simulink model "secondpart"  (R2022a)
settings: Solver=FixedStepAuto  StartTime=0.0  StopTime=5  FixedStep=0.2  RelTol=1e-3
settings Model: Creator=P1oruN7  LastModifiedBy=P1oruN7

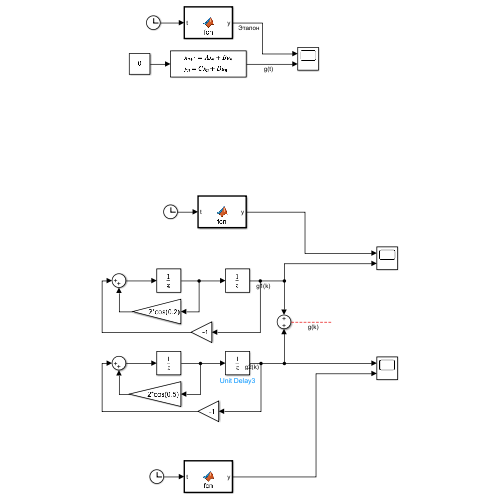
[thumbnail: Simulink's stored preview of the top-level diagram]
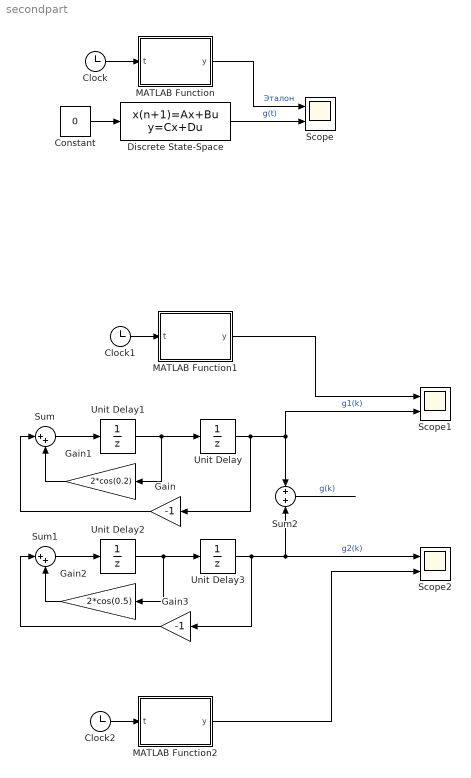
== system secondpart ==
  Clock : Clock
  Clock1 : Clock
  Clock2 : Clock
  Constant : Constant  Value=0
  Discrete State-Space : DiscreteStateSpace  A=[0 1 0 0; -1 2*cos(0.2) 0 0; 0 0 0 1; 0 0 -1 2*cos(0.5)]  B=[1; 1; 1; 1]  C=[1 0 1 0]  D=0  InitialCondition=[0; 8*sin(0.2); 1.5; 1.5*cos(0.5)]  SampleTime=0.2
  Gain : Gain  Gain=-1
  Gain1 : Gain  Gain=2*cos(0.2)
  Gain2 : Gain  Gain=2*cos(0.5)
  Gain3 : Gain  Gain=-1
  MATLAB Function : MATLAB Function  TreatAsAtomicUnit=on
  MATLAB Function1 : MATLAB Function  TreatAsAtomicUnit=on
  MATLAB Function2 : MATLAB Function  TreatAsAtomicUnit=on
  Scope : Scope  NumInputPorts=2
  Scope1 : Scope  NumInputPorts=2
  Scope2 : Scope  NumInputPorts=2
  Sum : Sum  Inputs=|++
  Sum1 : Sum  Inputs=|++
  Sum2 : Sum
  Unit Delay : UnitDelay  SampleTime=-1  HasFrameUpgradeWarning=on
  Unit Delay1 : UnitDelay  InitialCondition=8*sin(0.2)  SampleTime=-1  HasFrameUpgradeWarning=on
  Unit Delay2 : UnitDelay  InitialCondition=1.5*cos(0.5)  SampleTime=-1  HasFrameUpgradeWarning=on
  Unit Delay3 : UnitDelay  SampleTime=-1  HasFrameUpgradeWarning=on
  wires:
  Clock/1 -> MATLAB Function/1(t)
  Constant/1 -> Discrete State-Space/1
  Discrete State-Space/1 -> Scope/2  "g(t)"
  MATLAB Function/1(y) -> Scope/1  "Эталон"
  Sum2/1 -> ?  "g(k)"
  Unit Delay3/1 -> Gain3/1, Sum2/2, Scope2/1  "g2(k)"
  Unit Delay2/1 -> Gain2/1, Unit Delay3/1
  Gain2/1 -> Sum1/2
  Sum1/1 -> Unit Delay2/1
  Sum/1 -> Unit Delay1/1
  Gain1/1 -> Sum/2
  Gain/1 -> Sum/1
  Gain3/1 -> Sum1/1
  Unit Delay/1 -> Sum2/1, Scope1/2, Gain/1  "g1(k)"
  Unit Delay1/1 -> Unit Delay/1, Gain1/1
  Clock1/1 -> MATLAB Function1/1(t)
  MATLAB Function1/1(y) -> Scope1/1
  Clock2/1 -> MATLAB Function2/1(t)
  MATLAB Function2/1(y) -> Scope2/2

== matlab function secondpart/MATLAB Function ==
  data: t input; y output
function y = fcn(t)

y = 8*sin(t)+1.5*cos(2.5*t);

== matlab function secondpart/MATLAB Function2 ==
  data: t input; y output
function y = fcn(t)

y = 1.5*cos(2.5*t);

== matlab function secondpart/MATLAB Function1 ==
  data: t input; y output
function y = fcn(t)

y = 8*sin(t);
